simulink model "Intergration"  (R2018b)
settings: Solver=FixedStepDiscrete  StartTime=0.0  StopTime=inf  FixedStep=0.005  RelTol=1e-3
PostLoadFcn:
  | if any(exist('dsrtsu_mdlpostloadfcn', 'file') ~= 0), dsrtsu_mdlpostloadfcn('Execute', bdroot); end
values from neighbouring files (symbols this model uses):
  P_x165_On = 1.0    [CAN_Tx.sldd]
  P_x242_On = 1.0    [CAN_Tx.sldd]
  P_x246_On = 1.0    [CAN_Tx.sldd]
libraries: rtican x112, simulink x59
(part 27 of 31)

== system Intergration/TX/YRS1_0x131 ==
  <VehDynYawRate> : Inport
  In2 : Inport  Port=2
  Cast To Double{1..4} (4 alike) : DataTypeConversion  OutDataTypeStr=double
  Constant : Constant  Value=0  OutDataTypeStr=uint8
  Constant2 : Constant  Value=0  OutDataTypeStr=double
  Constant6 : Constant  Value=7  OutDataTypeStr=uint8
  RollingCounter1 : Subsystem
  S-Function Builder1 : S-Function  InitFcn=try, set_param(gcb,'FunctionName','CheckSum_Tx_Radar410'), end  FunctionName=CheckSum_Tx_Radar410  SFunctionModules=CheckSum_Tx_Radar410_wrapper  SFunctionDeploymentMode=off  EnableBusSupport=off  mask(S-Function Builder){}
      mask help: Simulink:masks:SFunctionBuilder_MD
      mask init: same as Intergration/Tx_410_10ms/S-Function Builder1
      settings: CopyFcn=set_param(gcbh,'LinkStatus','none')  PreSaveFcn=try, set_param(gcb,'FunctionName','CheckSum_Tx_Radar410'), end  OpenFcn=sfunctionwizard(gcbh)
      mask Display: plot(val(:,1),val(:,2)),disp(sys), port_label('input',1,'data'), port_label('input',2,'length'), port_label('output',1,'u8_crc8')
  Subsystem : Subsystem
  Subsystem1 : Subsystem
  Subsystem4 : Subsystem
  Vector Concatenate1 : Concatenate  NumInputs=7
  YRS1 : rtican/RTICAN Transmit (TX)   Reserved1=[]  Reserved2=[]  Reserved3=[]  Reserved4=[]  SfcnMessage=[]  Msg_Struct=[]  BoardTypeNo=[]  BoardNo=[]  ChannelNo=[]  Parameters=[]  DialogFcn=[]  UnitName=[]  Revision=[]  UnitValues=[]  DSProperties=struct('RTI',struct('Version',uint32(5),'BlockType',struct('isSLSource',uint8(1),'isSLSink',uint8(1),'isHWSource',uint8(0),'isHWSink',uint8(0),'isSetup',uint8(0),'isInline',uint8(1),'isNonInline',uint8(0),'isInterrupt',uint8(0),'isChannelwise',uint8(0)),'IOBoardType','RTICAN','UnitType','MESSAGE','Identifier','TX','DialogType','MSVC','BlockSet','RTICAN','SlaveProcessor','CAN'))  RTIBlockInterface=struct('InputPortsWidth',int32([1 1 1 1 1 1]),'InputPortsActive',[1 1 1 1 1 1],'InputPortsName',{{'YRS1_AliveCounter','YRS_YawRate','YRS_LateralAcce','YRS_YawRateSensorState','YRS_LateralSensorState','YRS1_Checksum'}},'InputPortsDataType',{{'SS_DOUBLE','SS_DOUBLE','SS_DOUBLE','SS_DOUBLE','SS_DOUBLE','SS_DOUBLE'}},'OutputPortsWidth',int32([1 1 1 1]),'OutputPortsActive',[1 1 1 1],'OutputPortsName',{{['TX status'],['TX time'],['TX delta time'],['TX delay time']}},'DialogFcn','rtican_message_interface_gui','BlockDisplay',{{'','center'}},'IconTransparency','on','InitLevel',3,'BlockName',struct('Token',{{'YRS1'}}),'SampleTime',{{-1}},'TriggerPort',{{'none'}},'EnablePort',{{'none'}})  RTIBlockParameters=struct('BoardTypeNo',{{1,'OFF',[]}},'BoardNo',{{3,'ON',[1 16]}},'ChannelNo',{{2,'ON',[1 2]}},'Parameters',{{struct('DataFileSupport',struct('DataFileSelectedMaster',1,'DataFileSelectedLocal',1,'DataFileName','c:\users\administrator.zx-201607042142\documents\matlab\zone\dbc\ars410od_privatecan.dbc|c:\users\administrator.zx-201607042142\desktop\zone\2020_demo\410\asr410od_public_can.dbc|','DataFileDate',{{{''},{['30-十一月-2020 09:38:41']}}},'SelectedFile','..\..\..\..\..\desktop\zone\2020_demo\410\asr410od_public_can.dbc','InterfaceFcn','rtican_dbc_file_parser'),'Options',struct('StatusSelected',1,'TimeSelected',1,'DeltaTimeSelected',1,'DelayTimeSelected',1,'DelayTimeTXCommandSelected',0,'EncodeSetUnusedBitsToOne',0,'EnableMsgLoopback',0,'TriggerPort',struct('Selected',0,'TriggerType',0),'EnablePortSelected',0,'SignalOnPortnameSelected',1,'UserCoding',struct('Selected',0,'InterfaceFile','UserEncodingFile','FcnName','UserEncodeFcn','InportSelected',0,'InportWidth',1,'OutportSelected',0,'OutportWidth',1),'TerminationMsg',struct('Selected',0,'Byte0_7','0'),'InitialMsg',struct('Selected',0,'Byte0_7','0')),'Message',struct('MsgOnBlocknameSelected',1,'MsgName','YRS1','MsgIdFormat',0,'MsgId',305,'MsgLength',8,'NumSignals',6,'SampleTime',-1,'StartTime',struct('Selected',0,'Value',3),'AutoRepeatTime',struct('Selected',0,'Value',0.1),'Timeout',struct('Selected',0,'Value',0.1),'DelayTime',struct('Selected',0,'Value',0.1),'Signal',struct('SgnName',{'YRS1_AliveCounter','YRS_YawRate','YRS_LateralAcce','YRS_YawRateSensorState','YRS_LateralSensorState','YRS1_Checksum'},'SgnStartBit',{0,16,32,49,51,56},'SgnLength',{4,16,16,2,2,8},'SgnType',{0,0,0,0,0,0},'ModeValue',{-1,-1,-1,-1,-1,-1},'DataType',{0,0,0,0,0,0},'ByteLayout',{2,2,2,2,2,2},'Factor',{1,0.01,0.001,1,1,1},'Offset',{0,-180,-2,0,0,0},'SgnComment',{{'YRS1_AliveCounter'},{'YRS_YawRate'},{'YRS_LateralAcce'},{'YRS_YawRateSensorState'},{'YRS_LateralSensorState'},{'YRS1_Checksum'}},'SgnUnit',{'','','','','',''},'Min',{0,-180,-2,0,0,0},'Max',{15,180,2,3,3,255},'SLDataType',{'SS_DOUBLE','SS_DOUBLE','SS_DOUBLE','SS_DOUBLE','SS_DOUBLE','SS_DOUBLE'}),'MsgIdNumFormat',1,'MsgComment',{{''}}),'Version',1.2,'general',struct('isFromLib',0)),'OFF',[]}},'GroupId',{{struct('Group',{{'RTICAN'}},'No',3,'Behavior',{{'NAMECHANGE'}},'BlockType',{{'SINK'}},'NameChangeFlag',0),'OFF',[]}},'SFcnRTICANMessage',{{struct('MsgType','TX','SFcnPortType','Scalar','MsgName','YRS1','MsgIdFormat','STD','MsgId',305,'MsgLength',8,'NumSignals',6,'SampleTime',-1,'StartTime',struct('Selected','no','Value',3),'AutoRepeatTime',struct('Selected','no','Value',0.1),'Timeout',struct('Selected','no','Value',0.1),'Signal',struct('SgnName',{'YRS1_AliveCounter','YRS_YawRate','YRS_LateralAcce','YRS_YawRateSensorState','YRS_LateralSensorState','YRS1_Checksum'},'SgnStartBit',{0,16,32,49,51,56},'SgnLength',{4,16,16,2,2,8},'SgnType',{'standard','standard','standard','standard','standard','standard'},'ModeValue',{-1,-1,-1,-1,-1,-1},'DataType',{['unsigned int'],['unsigned int'],['unsigned int'],['unsigned int'],['unsigned int'],['unsigned int']},'ByteLayout',{['motorola back.'],['motorola back.'],['motorola back.'],['motorola back.'],['motorola back.'],['motorola back.']},'Factor',{1,0.01,0.001,1,1,1},'Offset',{0,-180,-2,0,0,0},'SLDataType',{'SS_DOUBLE','SS_DOUBLE','SS_DOUBLE','SS_DOUBLE','SS_DOUBLE','SS_DOUBLE'}),'StatusSelected','yes','TimeSelected','yes','DeltaTimeSelected','yes','DelayTimeSelected','yes','DelayTimeTXCommandSelected','no','EncodeSetUnusedBitsToOne','no','EnableMsgLoopback','no','TriggerPort',struct('Selected','no','TriggerType',0),'EnablePortSelected','no','UserCoding',struct('Selected','no','InterfaceFile','UserEncodingFile','FcnName','UserEncodeFcn','InportSelected','no','InportWidth',1,'OutportSelected','no','OutportWidth',1),'TerminationMsg',struct('Selected','no','Byte0','0x00','Byte1','0x00','Byte2','0x00','Byte3','0x00','Byte4','0x00','Byte5','0x00','Byte6','0x00','Byte7','0x00'),'InitialMsg',struct('Selected','no','Byte0','0x00','Byte1','0x00','Byte2','0x00','Byte3','0x00','Byte4','0x00','Byte5','0x00','Byte6','0x00','Byte7','0x00'),'BoardType','DS1','BoardNo',3,'ControllerNo',2),'OFF',[]}},'TLCFileName',{{'rtican_tx_message','OFF',[]}})  RTISFcnParameters=struct('SFcnRTICANMessage','struct','TLCFileName','char')  RTIBlockParaDefault=struct('BoardTypeNo',4302,'BoardNo',1,'ChannelNo',1,'Parameters',struct('DataFileSupport',struct('DataFileSelectedMaster',0,'DataFileSelectedLocal',0,'DataFileName','','DataFileDate','','SelectedFile',['<no file selected>']),'Options',struct('StatusSelected',1,'TimeSelected',1,'DeltaTimeSelected',1,'DelayTimeSelected',1,'DelayTimeTXCommandSelected',0,'EncodeSetUnusedBitsToOne',0,'EnableMsgLoopback',0,'TriggerPort',struct('Selected',0,'TriggerType','rising'),'EnablePortSelected',0,'SignalOnPortnameSelected',1,'UserCoding',struct('Selected',0,'InterfaceFile','UserEncodingFile','FcnName','UserEncodeFcn','InportSelected',0,'InportWidth',1,'OutportSelected',0,'OutportWidth',1),'TerminationMsg',struct('Selected',0,'Byte0_7','0'),'InitialMsg',struct('Selected',0,'Byte0_7','0')),'Message',struct('MsgOnBlocknameSelected',0,'MsgName',['TX Message'],'MsgIdFormat',0,'MsgId',100,'MsgLength',8,'NumSignals',1,'SampleTime',-1,'StartTime',struct('Selected',0,'Value',0),'AutoRepeatTime',struct('Selected',0,'Value',0.1),'Timeout',struct('Selected',0,'Value',0.1),'DelayTime',struct('Selected',0,'Value',0.1),'Signal',struct('SgnName',['TX signal'],'SgnStartBit',0,'SgnLength',8,'SgnType',0,'ModeValue',-1,'DataType',0,'SLDataType','SS_DOUBLE','ByteLayout',0,'Factor',1,'Offset',0,'Min',0,'Max',255,'SgnComment',{{}},'SgnUnit',''),'MsgIdNumFormat',0,'MsgComment',{{''}}),'Version',1.2,'general',struct('isFromLib',1)),'GroupId',struct('Group',{{'RTICAN'}},'No',1,'Behavior',{{'NAMECHANGE'}},'BlockType',{{'SINK'}},'NameChangeFlag',0),'SFcnRTICANMessage',struct('MsgType','TX','MsgName',['TX Message'],'MsgIdFormat','STD','MsgId',100,'MsgLength',2,'NumSignals',1,'SampleTime',-1,'StartTime',struct('Selected','no','Value',0),'AutoRepeatTime',struct('Selected','no','Value',0.1),'Timeout',struct('Selected','no','Value',0.1),'DelayTime',struct('Selected','no','Value',0.1),'Signal',struct('SgnName',['TX signal'],'SgnStartBit',0,'SgnLength',8,'SgnType','standard','ModeValue',-1,'DataType',['unsigned int'],'ByteLayout',['little endian'],'SLDataType','SS_DOUBLE','Factor',1,'Offset',0),'StatusSelected','yes','TimeSelected','yes','DeltaTimeSelected','yes','DelayTimeSelected','yes','EnablePortSelected','no','EnableMsgLoopback','no','DelayTimeTXCommandSelected','no','EncodeSetUnusedBitsToOne','no','UserCoding',struct('Selected','no','InterfaceFile','UserDecodingFile','FcnName','UserDecodeFcn','InportSelected','no','InportWidth',1,'OutportSelected','no','OutportWidth',1),'TerminationMsg',struct('Selected','no','Byte0','0x00','Byte1','0x00','Byte2','0x00','Byte3','0x00','Byte4','0x00','Byte5','0x00','Byte6','0x00','Byte7','0x00'),'InitialMsg',struct('Selected','no','Byte0','0x00','Byte1','0x00','Byte2','0x00','Byte3','0x00','Byte4','0x00','Byte5','0x00','Byte6','0x00','Byte7','0x00'),'TriggerPort',struct('Selected','no','TriggerType','rising'),'BoardType','DS4302','BoardNo',1,'ControllerNo',1,'SFcnPortType','Scalar'),'TLCFileName','rtican_tx_message')
      settings: AttributesFormatString=Group Id: RTICAN3\n  SourceProductName=dSPACE RTI CAN Blockset
  wires:
  Subsystem1/1(Byte4) -> Vector Concatenate1/3
  Subsystem1/3(Byte5) -> Vector Concatenate1/4
  Subsystem/3(Byte3) -> Vector Concatenate1/2
  Subsystem/1(Byte2) -> Vector Concatenate1/1
  Constant2/1 -> YRS1/5, YRS1/4
  Subsystem1/2(Out2) -> Cast To Double3/1
  Cast To Double2/1 -> YRS1/6
  RollingCounter1/1(RC) -> Cast To Double4/1, Subsystem4/1(In1)
  Cast To Double4/1 -> YRS1/1
  Subsystem4/1(Byte6) -> Vector Concatenate1/5
  Cast To Double1/1 -> YRS1/3
  Constant6/1 -> S-Function Builder1/2
  Cast To Double3/1 -> YRS1/2
  Subsystem/2(Out2) -> Cast To Double1/1
  S-Function Builder1/1 -> Cast To Double2/1
  Vector Concatenate1/1 -> S-Function Builder1/1
  <VehDynYawRate>/1 -> Subsystem1/1(In1)
  In2/1 -> Subsystem/1(In1)
  Constant/1 -> Vector Concatenate1/7, Vector Concatenate1/6

== system Intergration/TX/YRS2_0x132 ==
  In1 : Inport
  Cast To Double1 : DataTypeConversion  OutDataTypeStr=double
  Cast To Double2 : DataTypeConversion  OutDataTypeStr=double
  Cast To Double3 : DataTypeConversion  OutDataTypeStr=double
  Constant : Constant  Value=0  OutDataTypeStr=uint8
  Constant1 : Constant  Value=0  OutDataTypeStr=double
  Constant6 : Constant  Value=7  OutDataTypeStr=uint8
  RollingCounter1 : Subsystem
  S-Function Builder1 : S-Function  InitFcn=try, set_param(gcb,'FunctionName','CheckSum_Tx_Radar410'), end  FunctionName=CheckSum_Tx_Radar410  SFunctionModules=CheckSum_Tx_Radar410_wrapper  SFunctionDeploymentMode=off  EnableBusSupport=off  mask(S-Function Builder){}
      mask help: Simulink:masks:SFunctionBuilder_MD
      mask init: same as Intergration/Tx_410_10ms/S-Function Builder1
      settings: CopyFcn=set_param(gcbh,'LinkStatus','none')  PreSaveFcn=try, set_param(gcb,'FunctionName','CheckSum_Tx_Radar410'), end  OpenFcn=sfunctionwizard(gcbh)
      mask Display: plot(val(:,1),val(:,2)),disp(sys), port_label('input',1,'data'), port_label('input',2,'length'), port_label('output',1,'u8_crc8')
  Subsystem : Subsystem
  Subsystem4 : Subsystem
  Vector Concatenate1 : Concatenate  NumInputs=7
  YRS2 : rtican/RTICAN Transmit (TX)   Reserved1=[]  Reserved2=[]  Reserved3=[]  Reserved4=[]  SfcnMessage=[]  Msg_Struct=[]  BoardTypeNo=[]  BoardNo=[]  ChannelNo=[]  Parameters=[]  DialogFcn=[]  UnitName=[]  Revision=[]  UnitValues=[]  DSProperties=struct('RTI',struct('Version',uint32(5),'BlockType',struct('isSLSource',uint8(1),'isSLSink',uint8(1),'isHWSource',uint8(0),'isHWSink',uint8(0),'isSetup',uint8(0),'isInline',uint8(1),'isNonInline',uint8(0),'isInterrupt',uint8(0),'isChannelwise',uint8(0)),'IOBoardType','RTICAN','UnitType','MESSAGE','Identifier','TX','DialogType','MSVC','BlockSet','RTICAN','SlaveProcessor','CAN'))  RTIBlockInterface=struct('InputPortsWidth',int32([1 1 1 1]),'InputPortsActive',[1 1 1 1],'InputPortsName',{{'YRS_AliveCounter','YRS_LongitAcce','YRS_LongitSensorState','YRS2_Checksum'}},'InputPortsDataType',{{'SS_DOUBLE','SS_DOUBLE','SS_DOUBLE','SS_DOUBLE'}},'OutputPortsWidth',int32([1 1 1 1]),'OutputPortsActive',[1 1 1 1],'OutputPortsName',{{['TX status'],['TX time'],['TX delta time'],['TX delay time']}},'DialogFcn','rtican_message_interface_gui','BlockDisplay',{{'','center'}},'IconTransparency','on','InitLevel',3,'BlockName',struct('Token',{{'YRS2'}}),'SampleTime',{{-1}},'TriggerPort',{{'none'}},'EnablePort',{{'none'}})  RTIBlockParameters=struct('BoardTypeNo',{{1,'OFF',[]}},'BoardNo',{{3,'ON',[1 16]}},'ChannelNo',{{2,'ON',[1 2]}},'Parameters',{{struct('DataFileSupport',struct('DataFileSelectedMaster',1,'DataFileSelectedLocal',1,'DataFileName','c:\users\administrator.zx-201607042142\documents\matlab\zone\dbc\ars410od_privatecan.dbc|c:\users\administrator.zx-201607042142\desktop\zone\2020_demo\410\asr410od_public_can.dbc|','DataFileDate',{{{''},{['30-十一月-2020 09:38:41']}}},'SelectedFile','..\..\..\..\..\desktop\zone\2020_demo\410\asr410od_public_can.dbc','InterfaceFcn','rtican_dbc_file_parser'),'Options',struct('StatusSelected',1,'TimeSelected',1,'DeltaTimeSelected',1,'DelayTimeSelected',1,'DelayTimeTXCommandSelected',0,'EncodeSetUnusedBitsToOne',0,'EnableMsgLoopback',0,'TriggerPort',struct('Selected',0,'TriggerType',0),'EnablePortSelected',0,'SignalOnPortnameSelected',1,'UserCoding',struct('Selected',0,'InterfaceFile','UserEncodingFile','FcnName','UserEncodeFcn','InportSelected',0,'InportWidth',1,'OutportSelected',0,'OutportWidth',1),'TerminationMsg',struct('Selected',0,'Byte0_7','0'),'InitialMsg',struct('Selected',0,'Byte0_7','0')),'Message',struct('MsgOnBlocknameSelected',1,'MsgName','YRS2','MsgIdFormat',0,'MsgId',306,'MsgLength',8,'NumSignals',4,'SampleTime',-1,'StartTime',struct('Selected',0,'Value',3),'AutoRepeatTime',struct('Selected',0,'Value',0.1),'Timeout',struct('Selected',0,'Value',0.1),'DelayTime',struct('Selected',0,'Value',0.1),'Signal',struct('SgnName',{'YRS_AliveCounter','YRS_LongitAcce','YRS_LongitSensorState','YRS2_Checksum'},'SgnStartBit',{0,32,54,56},'SgnLength',{4,16,2,8},'SgnType',{0,0,0,0},'ModeValue',{-1,-1,-1,-1},'DataType',{0,0,0,0},'ByteLayout',{2,2,2,2},'Factor',{1,0.001,1,1},'Offset',{0,-2,0,0},'SgnComment',{{'YRS_AliveCounter'},{'YRS_LongitAcce'},{'YRS_LongitSensorState'},{'YRS2_Checksum'}},'SgnUnit',{'','','',''},'Min',{0,-2,0,0},'Max',{15,2,3,255},'SLDataType',{'SS_DOUBLE','SS_DOUBLE','SS_DOUBLE','SS_DOUBLE'}),'MsgIdNumFormat',1,'MsgComment',{{''}}),'Version',1.2,'general',struct('isFromLib',0)),'OFF',[]}},'GroupId',{{struct('Group',{{'RTICAN'}},'No',3,'Behavior',{{'NAMECHANGE'}},'BlockType',{{'SINK'}},'NameChangeFlag',0),'OFF',[]}},'SFcnRTICANMessage',{{struct('MsgType','TX','SFcnPortType','Scalar','MsgName','YRS2','MsgIdFormat','STD','MsgId',306,'MsgLength',8,'NumSignals',4,'SampleTime',-1,'StartTime',struct('Selected','no','Value',3),'AutoRepeatTime',struct('Selected','no','Value',0.1),'Timeout',struct('Selected','no','Value',0.1),'Signal',struct('SgnName',{'YRS_AliveCounter','YRS_LongitAcce','YRS_LongitSensorState','YRS2_Checksum'},'SgnStartBit',{0,32,54,56},'SgnLength',{4,16,2,8},'SgnType',{'standard','standard','standard','standard'},'ModeValue',{-1,-1,-1,-1},'DataType',{['unsigned int'],['unsigned int'],['unsigned int'],['unsigned int']},'ByteLayout',{['motorola back.'],['motorola back.'],['motorola back.'],['motorola back.']},'Factor',{1,0.001,1,1},'Offset',{0,-2,0,0},'SLDataType',{'SS_DOUBLE','SS_DOUBLE','SS_DOUBLE','SS_DOUBLE'}),'StatusSelected','yes','TimeSelected','yes','DeltaTimeSelected','yes','DelayTimeSelected','yes','DelayTimeTXCommandSelected','no','EncodeSetUnusedBitsToOne','no','EnableMsgLoopback','no','TriggerPort',struct('Selected','no','TriggerType',0),'EnablePortSelected','no','UserCoding',struct('Selected','no','InterfaceFile','UserEncodingFile','FcnName','UserEncodeFcn','InportSelected','no','InportWidth',1,'OutportSelected','no','OutportWidth',1),'TerminationMsg',struct('Selected','no','Byte0','0x00','Byte1','0x00','Byte2','0x00','Byte3','0x00','Byte4','0x00','Byte5','0x00','Byte6','0x00','Byte7','0x00'),'InitialMsg',struct('Selected','no','Byte0','0x00','Byte1','0x00','Byte2','0x00','Byte3','0x00','Byte4','0x00','Byte5','0x00','Byte6','0x00','Byte7','0x00'),'BoardType','DS1','BoardNo',3,'ControllerNo',2),'OFF',[]}},'TLCFileName',{{'rtican_tx_message','OFF',[]}})  RTISFcnParameters=struct('SFcnRTICANMessage','struct','TLCFileName','char')  RTIBlockParaDefault=struct('BoardTypeNo',4302,'BoardNo',1,'ChannelNo',1,'Parameters',struct('DataFileSupport',struct('DataFileSelectedMaster',0,'DataFileSelectedLocal',0,'DataFileName','','DataFileDate','','SelectedFile',['<no file selected>']),'Options',struct('StatusSelected',1,'TimeSelected',1,'DeltaTimeSelected',1,'DelayTimeSelected',1,'DelayTimeTXCommandSelected',0,'EncodeSetUnusedBitsToOne',0,'EnableMsgLoopback',0,'TriggerPort',struct('Selected',0,'TriggerType','rising'),'EnablePortSelected',0,'SignalOnPortnameSelected',1,'UserCoding',struct('Selected',0,'InterfaceFile','UserEncodingFile','FcnName','UserEncodeFcn','InportSelected',0,'InportWidth',1,'OutportSelected',0,'OutportWidth',1),'TerminationMsg',struct('Selected',0,'Byte0_7','0'),'InitialMsg',struct('Selected',0,'Byte0_7','0')),'Message',struct('MsgOnBlocknameSelected',0,'MsgName',['TX Message'],'MsgIdFormat',0,'MsgId',100,'MsgLength',8,'NumSignals',1,'SampleTime',-1,'StartTime',struct('Selected',0,'Value',0),'AutoRepeatTime',struct('Selected',0,'Value',0.1),'Timeout',struct('Selected',0,'Value',0.1),'DelayTime',struct('Selected',0,'Value',0.1),'Signal',struct('SgnName',['TX signal'],'SgnStartBit',0,'SgnLength',8,'SgnType',0,'ModeValue',-1,'DataType',0,'SLDataType','SS_DOUBLE','ByteLayout',0,'Factor',1,'Offset',0,'Min',0,'Max',255,'SgnComment',{{}},'SgnUnit',''),'MsgIdNumFormat',0,'MsgComment',{{''}}),'Version',1.2,'general',struct('isFromLib',1)),'GroupId',struct('Group',{{'RTICAN'}},'No',1,'Behavior',{{'NAMECHANGE'}},'BlockType',{{'SINK'}},'NameChangeFlag',0),'SFcnRTICANMessage',struct('MsgType','TX','MsgName',['TX Message'],'MsgIdFormat','STD','MsgId',100,'MsgLength',2,'NumSignals',1,'SampleTime',-1,'StartTime',struct('Selected','no','Value',0),'AutoRepeatTime',struct('Selected','no','Value',0.1),'Timeout',struct('Selected','no','Value',0.1),'DelayTime',struct('Selected','no','Value',0.1),'Signal',struct('SgnName',['TX signal'],'SgnStartBit',0,'SgnLength',8,'SgnType','standard','ModeValue',-1,'DataType',['unsigned int'],'ByteLayout',['little endian'],'SLDataType','SS_DOUBLE','Factor',1,'Offset',0),'StatusSelected','yes','TimeSelected','yes','DeltaTimeSelected','yes','DelayTimeSelected','yes','EnablePortSelected','no','EnableMsgLoopback','no','DelayTimeTXCommandSelected','no','EncodeSetUnusedBitsToOne','no','UserCoding',struct('Selected','no','InterfaceFile','UserDecodingFile','FcnName','UserDecodeFcn','InportSelected','no','InportWidth',1,'OutportSelected','no','OutportWidth',1),'TerminationMsg',struct('Selected','no','Byte0','0x00','Byte1','0x00','Byte2','0x00','Byte3','0x00','Byte4','0x00','Byte5','0x00','Byte6','0x00','Byte7','0x00'),'InitialMsg',struct('Selected','no','Byte0','0x00','Byte1','0x00','Byte2','0x00','Byte3','0x00','Byte4','0x00','Byte5','0x00','Byte6','0x00','Byte7','0x00'),'TriggerPort',struct('Selected','no','TriggerType','rising'),'BoardType','DS4302','BoardNo',1,'ControllerNo',1,'SFcnPortType','Scalar'),'TLCFileName','rtican_tx_message')
      settings: AttributesFormatString=Group Id: RTICAN3\n  SourceProductName=dSPACE RTI CAN Blockset
  wires:
  In1/1 -> Subsystem/1(In1)
  Constant6/1 -> S-Function Builder1/2
  Subsystem/1(Byte2) -> Vector Concatenate1/1
  Cast To Double2/1 -> YRS2/2
  RollingCounter1/1(RC) -> Subsystem4/1(In1), Cast To Double1/1
  Subsystem/3(Byte3) -> Vector Concatenate1/2
  Vector Concatenate1/1 -> S-Function Builder1/1
  Cast To Double1/1 -> YRS2/1
  Cast To Double3/1 -> YRS2/4
  Subsystem/2(Out2) -> Cast To Double2/1
  Constant1/1 -> YRS2/3
  Subsystem4/1(Byte6) -> Vector Concatenate1/3
  S-Function Builder1/1 -> Cast To Double3/1
  Constant/1 -> Vector Concatenate1/7, Vector Concatenate1/6, Vector Concatenate1/5, Vector Concatenate1/4

== system Intergration/Tx_410_10ms/RollingCounter1 ==
  Add2 : Sum
  Constant5 : Constant
  Constant6 : Constant  Value=-1
  Delay : Delay  DelayLength=1
  Switch : Switch  Criteria=u2 > Threshold  Threshold=14
  RC : Outport
  wires:
  Constant6/1 -> Switch/1
  Switch/1 -> Add2/2
  Delay/1 -> RC/1, Switch/3, Switch/2
  Add2/1 -> Delay/1
  Constant5/1 -> Add2/1

== system Intergration/Tx_410_10ms/Subsystem ==
  In1 : Inport
  Bitwise Operator1 : simulink/Logic and Bit Operations/Bitwise Operator  logicop=AND  UseBitMask=on  BitMask=bin2dec('11111111')  BitMaskRealWorld=Stored Integer
  Data Type Conversion1 : DataTypeConversion  OutDataTypeStr=uint8
  Byte2 : Outport
  wires:
  Data Type Conversion1/1 -> Bitwise Operator1/1
  Bitwise Operator1/1 -> Byte2/1
  In1/1 -> Data Type Conversion1/1

== system Intergration/Tx_410_10ms/Subsystem1 ==
  In1 : Inport
  Add : Sum
  Add1 : Sum  Inputs=+-
  Bitwise Operator1 : simulink/Logic and Bit Operations/Bitwise Operator  logicop=AND  UseBitMask=on  BitMask=bin2dec('11111111')  BitMaskRealWorld=Stored Integer
  Bitwise Operator2 : simulink/Logic and Bit Operations/Bitwise Operator  logicop=AND  UseBitMask=on  BitMask=bin2dec('11111111')  BitMaskRealWorld=Stored Integer
  Constant1 : Constant  Value=780
  Constant2 : Constant  Value=0.1
  Constant3 : Constant  Value=0.1
  Constant4 : Constant  Value=780
  Data Type Conversion1 : DataTypeConversion  OutDataTypeStr=uint16
  Data Type Conversion2 : DataTypeConversion  OutDataTypeStr=uint8
  Data Type Conversion3 : DataTypeConversion  OutDataTypeStr=uint8
  Divide1 : Product  Inputs=*/
  Multiply : Product
  Shift Arithmetic1 : ArithShift  BitShiftNumber=8  BitShiftDirection=Right
  Byte0 : Outport
  Out2 : Outport  Port=2
  Byte1 : Outport  Port=3
  wires:
  Constant2/1 -> Divide1/2
  Constant1/1 -> Add/2
  Data Type Conversion1/1 -> Bitwise Operator2/1, Multiply/1, Shift Arithmetic1/1
  Shift Arithmetic1/1 -> Bitwise Operator1/1
  Constant4/1 -> Add1/2
  Constant3/1 -> Multiply/2
  Multiply/1 -> Add1/1
  Bitwise Operator1/1 -> Data Type Conversion2/1
  Divide1/1 -> Data Type Conversion1/1
  Add/1 -> Divide1/1
  Add1/1 -> Out2/1
  Bitwise Operator2/1 -> Data Type Conversion3/1
  In1/1 -> Add/1
  Data Type Conversion2/1 -> Byte0/1
  Data Type Conversion3/1 -> Byte1/1

== system Intergration/Tx_410_10ms/Subsystem4 ==
  In1 : Inport
  Bitwise Operator2 : simulink/Logic and Bit Operations/Bitwise Operator  logicop=AND  UseBitMask=on  BitMask=bin2dec('11110000')  BitMaskRealWorld=Stored Integer
  Data Type Conversion1 : DataTypeConversion  OutDataTypeStr=uint8
  Shift Arithmetic1 : ArithShift  BitShiftNumber=4  BitShiftDirection=Left
  Byte4 : Outport
  wires:
  In1/1 -> Data Type Conversion1/1
  Bitwise Operator2/1 -> Byte4/1
  Data Type Conversion1/1 -> Shift Arithmetic1/1
  Shift Arithmetic1/1 -> Bitwise Operator2/1

== system Intergration/RTI Data/RTI Data Store/RTI Data Store ==
  RTI Data Store : Subsystem  mask(RTI_DATA_STORE){}
      mask help:
      | RTI Data Store Block. This block is used by RTI to store internal model dependent data. Deleting this block will result in data loss.
      |
      | NEVER DELETE, COPY, OR MODIFY THIS BLOCK!
      mask Help:
      | RTI Data Store Block. This block is used by RTI to store internal model dependent data. Deleting this block will result in data loss.
      | 
      | NEVER DELETE, COPY, OR MODIFY THIS BLOCK!
      mask Display: text(0.5, 0.5, ' ', 'HorizontalAlignment', 'center');

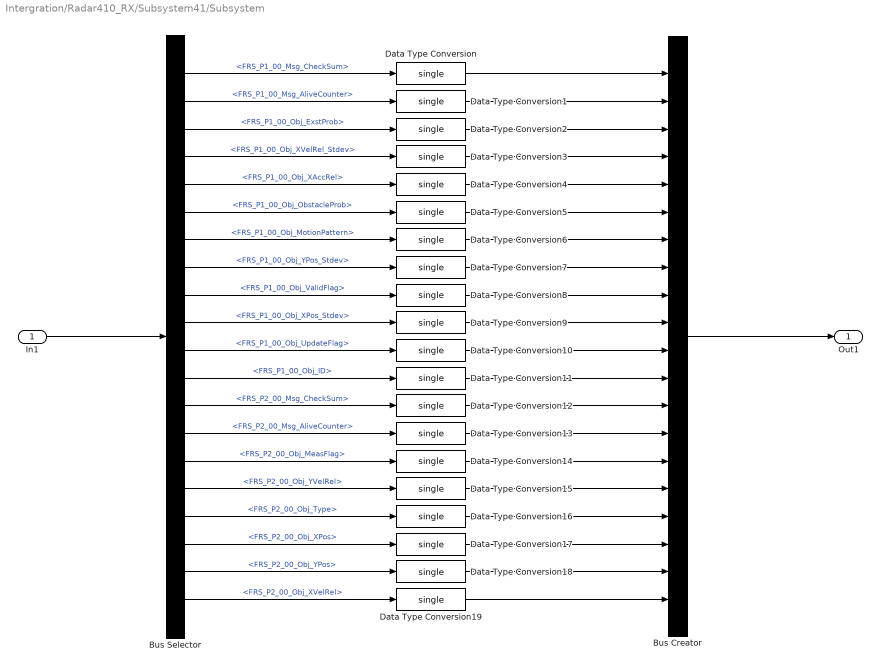
== system Intergration/Radar410_RX/Subsystem41/Subsystem ==
  In1 : Inport
  Bus Creator : BusCreator  Inputs=20  OutDataTypeStr=Bus: Obj_Data  NonVirtualBus=on
      settings: InheritFromInputs=off
  Bus Selector : BusSelector  OutputSignals=FRS_P1_00_Msg_CheckSum,FRS_P1_00_Msg_AliveCounter,FRS_P1_00_Obj_ExstProb,FRS_P1_00_Obj_XVelRel_Stdev,FRS_P1_00_Obj_XAccRel,FRS_P1_00_Obj_ObstacleProb,FRS_P1_00_Obj_MotionPattern,FRS_P1_00_Obj_YPos_Stdev,FRS_P1_00_Obj_ValidFlag,FRS_P1_00_Obj_XPos_Stdev,FRS_P1_00_Obj_UpdateFlag,FRS_P1_00_Obj_ID,FRS_P2_00_Msg_CheckSum,FRS_P2_00_Msg_AliveCounter,FRS_P2_00_Obj_MeasFlag,FRS_P2_00_Obj_YVelRel,FRS_P2_00_Obj_Type,FRS_P2_00_Obj_XPos,FRS_P2_00_Obj_YPos,FRS_P2_00_Obj_XVelRel
  Data Type Conversion{,1..19} (20 alike) : DataTypeConversion  OutDataTypeStr=single
  Out1 : Outport  OutDataTypeStr=Bus: Obj_Data
  wires:
  Data Type Conversion12/1 -> Bus Creator/13
  Bus Selector/5 -> Data Type Conversion4/1  "<FRS_P1_00_Obj_XAccRel>"
  Bus Selector/8 -> Data Type Conversion7/1  "<FRS_P1_00_Obj_YPos_Stdev>"
  Data Type Conversion15/1 -> Bus Creator/16
  Bus Selector/1 -> Data Type Conversion/1  "<FRS_P1_00_Msg_CheckSum>"
  Bus Selector/15 -> Data Type Conversion14/1  "<FRS_P2_00_Obj_MeasFlag>"
  Bus Selector/3 -> Data Type Conversion2/1  "<FRS_P1_00_Obj_ExstProb>"
  Bus Selector/13 -> Data Type Conversion12/1  "<FRS_P2_00_Msg_CheckSum>"
  Bus Selector/2 -> Data Type Conversion1/1  "<FRS_P1_00_Msg_AliveCounter>"
  Data Type Conversion11/1 -> Bus Creator/12
  Data Type Conversion5/1 -> Bus Creator/6
  Bus Selector/4 -> Data Type Conversion3/1  "<FRS_P1_00_Obj_XVelRel_Stdev>"
  Bus Selector/7 -> Data Type Conversion6/1  "<FRS_P1_00_Obj_MotionPattern>"
  Data Type Conversion9/1 -> Bus Creator/10
  Bus Selector/6 -> Data Type Conversion5/1  "<FRS_P1_00_Obj_ObstacleProb>"
  Data Type Conversion18/1 -> Bus Creator/19
  Bus Selector/11 -> Data Type Conversion10/1  "<FRS_P1_00_Obj_UpdateFlag>"
  Data Type Conversion17/1 -> Bus Creator/18
  Bus Selector/16 -> Data Type Conversion15/1  "<FRS_P2_00_Obj_YVelRel>"
  Data Type Conversion6/1 -> Bus Creator/7
  Bus Selector/12 -> Data Type Conversion11/1  "<FRS_P1_00_Obj_ID>"
  Data Type Conversion16/1 -> Bus Creator/17
  Bus Selector/9 -> Data Type Conversion8/1  "<FRS_P1_00_Obj_ValidFlag>"
  Bus Selector/17 -> Data Type Conversion16/1  "<FRS_P2_00_Obj_Type>"
  Bus Selector/10 -> Data Type Conversion9/1  "<FRS_P1_00_Obj_XPos_Stdev>"
  Data Type Conversion10/1 -> Bus Creator/11
  Bus Selector/14 -> Data Type Conversion13/1  "<FRS_P2_00_Msg_AliveCounter>"
  Bus Selector/19 -> Data Type Conversion18/1  "<FRS_P2_00_Obj_YPos>"
  Bus Selector/18 -> Data Type Conversion17/1  "<FRS_P2_00_Obj_XPos>"
  Bus Selector/20 -> Data Type Conversion19/1  "<FRS_P2_00_Obj_XVelRel>"
  In1/1 -> Bus Selector/1
  Bus Creator/1 -> Out1/1
  Data Type Conversion/1 -> Bus Creator/1
  Data Type Conversion2/1 -> Bus Creator/3
  Data Type Conversion13/1 -> Bus Creator/14
  Data Type Conversion1/1 -> Bus Creator/2
  Data Type Conversion4/1 -> Bus Creator/5
  Data Type Conversion3/1 -> Bus Creator/4
  Data Type Conversion7/1 -> Bus Creator/8
  Data Type Conversion8/1 -> Bus Creator/9
  Data Type Conversion14/1 -> Bus Creator/15
  Data Type Conversion19/1 -> Bus Creator/20

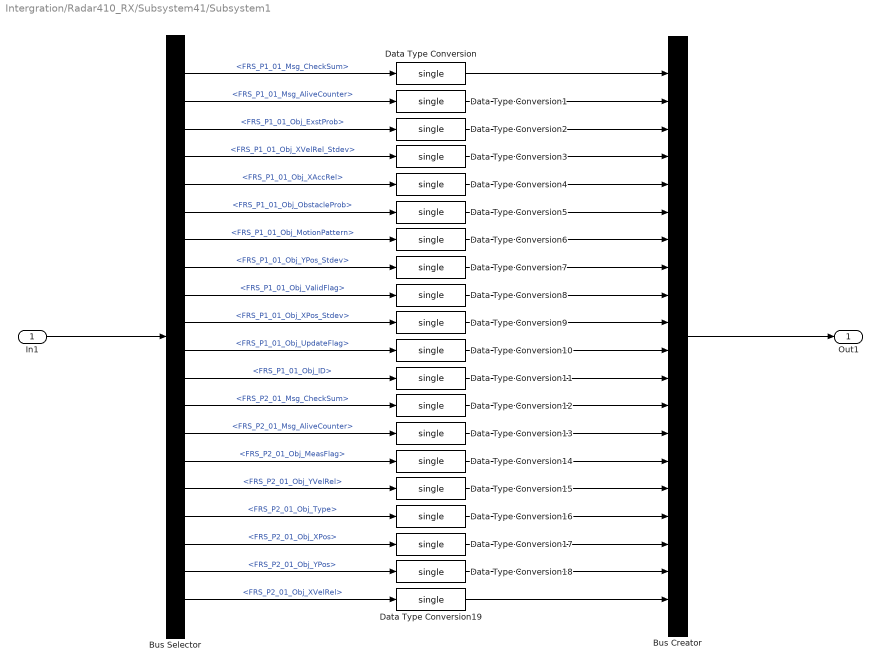
== system Intergration/Radar410_RX/Subsystem41/Subsystem1 ==
  In1 : Inport
  Bus Creator : BusCreator  Inputs=20  OutDataTypeStr=Bus: Obj_Data  NonVirtualBus=on
      settings: InheritFromInputs=off
  Bus Selector : BusSelector  OutputSignals=FRS_P1_01_Msg_CheckSum,FRS_P1_01_Msg_AliveCounter,FRS_P1_01_Obj_ExstProb,FRS_P1_01_Obj_XVelRel_Stdev,FRS_P1_01_Obj_XAccRel,FRS_P1_01_Obj_ObstacleProb,FRS_P1_01_Obj_MotionPattern,FRS_P1_01_Obj_YPos_Stdev,FRS_P1_01_Obj_ValidFlag,FRS_P1_01_Obj_XPos_Stdev,FRS_P1_01_Obj_UpdateFlag,FRS_P1_01_Obj_ID,FRS_P2_01_Msg_CheckSum,FRS_P2_01_Msg_AliveCounter,FRS_P2_01_Obj_MeasFlag,FRS_P2_01_Obj_YVelRel,FRS_P2_01_Obj_Type,FRS_P2_01_Obj_XPos,FRS_P2_01_Obj_YPos,FRS_P2_01_Obj_XVelRel
  Data Type Conversion{,1..19} (20 alike) : DataTypeConversion  OutDataTypeStr=single
  Out1 : Outport  OutDataTypeStr=Bus: Obj_Data
  wires:
  Data Type Conversion19/1 -> Bus Creator/20
  Data Type Conversion14/1 -> Bus Creator/15
  Data Type Conversion8/1 -> Bus Creator/9
  Data Type Conversion7/1 -> Bus Creator/8
  Data Type Conversion3/1 -> Bus Creator/4
  Data Type Conversion4/1 -> Bus Creator/5
  Data Type Conversion1/1 -> Bus Creator/2
  Data Type Conversion13/1 -> Bus Creator/14
  Data Type Conversion2/1 -> Bus Creator/3
  Data Type Conversion/1 -> Bus Creator/1
  Bus Creator/1 -> Out1/1
  In1/1 -> Bus Selector/1
  Bus Selector/20 -> Data Type Conversion19/1  "<FRS_P2_01_Obj_XVelRel>"
  Bus Selector/18 -> Data Type Conversion17/1  "<FRS_P2_01_Obj_XPos>"
  Bus Selector/19 -> Data Type Conversion18/1  "<FRS_P2_01_Obj_YPos>"
  Bus Selector/14 -> Data Type Conversion13/1  "<FRS_P2_01_Msg_AliveCounter>"
  Data Type Conversion10/1 -> Bus Creator/11
  Bus Selector/10 -> Data Type Conversion9/1  "<FRS_P1_01_Obj_XPos_Stdev>"
  Bus Selector/17 -> Data Type Conversion16/1  "<FRS_P2_01_Obj_Type>"
  Bus Selector/9 -> Data Type Conversion8/1  "<FRS_P1_01_Obj_ValidFlag>"
  Data Type Conversion16/1 -> Bus Creator/17
  Bus Selector/12 -> Data Type Conversion11/1  "<FRS_P1_01_Obj_ID>"
  Data Type Conversion6/1 -> Bus Creator/7
  Bus Selector/16 -> Data Type Conversion15/1  "<FRS_P2_01_Obj_YVelRel>"
  Data Type Conversion17/1 -> Bus Creator/18
  Bus Selector/11 -> Data Type Conversion10/1  "<FRS_P1_01_Obj_UpdateFlag>"
  Data Type Conversion18/1 -> Bus Creator/19
  Bus Selector/6 -> Data Type Conversion5/1  "<FRS_P1_01_Obj_ObstacleProb>"
  Data Type Conversion9/1 -> Bus Creator/10
  Bus Selector/7 -> Data Type Conversion6/1  "<FRS_P1_01_Obj_MotionPattern>"
  Bus Selector/4 -> Data Type Conversion3/1  "<FRS_P1_01_Obj_XVelRel_Stdev>"
  Data Type Conversion5/1 -> Bus Creator/6
  Data Type Conversion11/1 -> Bus Creator/12
  Bus Selector/2 -> Data Type Conversion1/1  "<FRS_P1_01_Msg_AliveCounter>"
  Bus Selector/13 -> Data Type Conversion12/1  "<FRS_P2_01_Msg_CheckSum>"
  Bus Selector/3 -> Data Type Conversion2/1  "<FRS_P1_01_Obj_ExstProb>"
  Bus Selector/15 -> Data Type Conversion14/1  "<FRS_P2_01_Obj_MeasFlag>"
  Bus Selector/1 -> Data Type Conversion/1  "<FRS_P1_01_Msg_CheckSum>"
  Data Type Conversion15/1 -> Bus Creator/16
  Bus Selector/8 -> Data Type Conversion7/1  "<FRS_P1_01_Obj_YPos_Stdev>"
  Bus Selector/5 -> Data Type Conversion4/1  "<FRS_P1_01_Obj_XAccRel>"
  Data Type Conversion12/1 -> Bus Creator/13

== system Intergration/Radar410_RX/Subsystem41/Subsystem10 ==
  In1 : Inport
  Bus Creator : BusCreator  Inputs=20  OutDataTypeStr=Bus: Obj_Data  NonVirtualBus=on
      settings: InheritFromInputs=off
  Bus Selector : BusSelector  OutputSignals=FRS_P1_10_Msg_CheckSum,FRS_P1_10_Msg_AliveCounter,FRS_P1_10_Obj_ExstProb,FRS_P1_10_Obj_XVelRel_Stdev,FRS_P1_10_Obj_XAccRel,FRS_P1_10_Obj_ObstacleProb,FRS_P1_10_Obj_MotionPattern,FRS_P1_10_Obj_YPos_Stdev,FRS_P1_10_Obj_ValidFlag,FRS_P1_10_Obj_XPos_Stdev,FRS_P1_10_Obj_UpdateFlag,FRS_P1_10_Obj_ID,FRS_P2_10_Msg_CheckSum,FRS_P2_10_Msg_AliveCounter,FRS_P2_10_Obj_MeasFlag,FRS_P2_10_Obj_YVelRel,FRS_P2_10_Obj_Type,FRS_P2_10_Obj_XPos,FRS_P2_10_Obj_YPos,FRS_P2_10_Obj_XVelRel
  Data Type Conversion{,1..19} (20 alike) : DataTypeConversion  OutDataTypeStr=single
  Out1 : Outport  OutDataTypeStr=Bus: Obj_Data
  wires:
  Data Type Conversion19/1 -> Bus Creator/20
  Data Type Conversion14/1 -> Bus Creator/15
  Data Type Conversion8/1 -> Bus Creator/9
  Data Type Conversion7/1 -> Bus Creator/8
  Data Type Conversion3/1 -> Bus Creator/4
  Data Type Conversion4/1 -> Bus Creator/5
  Data Type Conversion1/1 -> Bus Creator/2
  Data Type Conversion13/1 -> Bus Creator/14
  Data Type Conversion2/1 -> Bus Creator/3
  Data Type Conversion/1 -> Bus Creator/1
  Bus Creator/1 -> Out1/1
  In1/1 -> Bus Selector/1
  Bus Selector/20 -> Data Type Conversion19/1  "<FRS_P2_10_Obj_XVelRel>"
  Bus Selector/18 -> Data Type Conversion17/1  "<FRS_P2_10_Obj_XPos>"
  Bus Selector/19 -> Data Type Conversion18/1  "<FRS_P2_10_Obj_YPos>"
  Bus Selector/14 -> Data Type Conversion13/1  "<FRS_P2_10_Msg_AliveCounter>"
  Data Type Conversion10/1 -> Bus Creator/11
  Bus Selector/10 -> Data Type Conversion9/1  "<FRS_P1_10_Obj_XPos_Stdev>"
  Bus Selector/17 -> Data Type Conversion16/1  "<FRS_P2_10_Obj_Type>"
  Bus Selector/9 -> Data Type Conversion8/1  "<FRS_P1_10_Obj_ValidFlag>"
  Data Type Conversion16/1 -> Bus Creator/17
  Bus Selector/12 -> Data Type Conversion11/1  "<FRS_P1_10_Obj_ID>"
  Data Type Conversion6/1 -> Bus Creator/7
  Bus Selector/16 -> Data Type Conversion15/1  "<FRS_P2_10_Obj_YVelRel>"
  Data Type Conversion17/1 -> Bus Creator/18
  Bus Selector/11 -> Data Type Conversion10/1  "<FRS_P1_10_Obj_UpdateFlag>"
  Data Type Conversion18/1 -> Bus Creator/19
  Bus Selector/6 -> Data Type Conversion5/1  "<FRS_P1_10_Obj_ObstacleProb>"
  Data Type Conversion9/1 -> Bus Creator/10
  Bus Selector/7 -> Data Type Conversion6/1  "<FRS_P1_10_Obj_MotionPattern>"
  Bus Selector/4 -> Data Type Conversion3/1  "<FRS_P1_10_Obj_XVelRel_Stdev>"
  Data Type Conversion5/1 -> Bus Creator/6
  Data Type Conversion11/1 -> Bus Creator/12
  Bus Selector/2 -> Data Type Conversion1/1  "<FRS_P1_10_Msg_AliveCounter>"
  Bus Selector/13 -> Data Type Conversion12/1  "<FRS_P2_10_Msg_CheckSum>"
  Bus Selector/3 -> Data Type Conversion2/1  "<FRS_P1_10_Obj_ExstProb>"
  Bus Selector/15 -> Data Type Conversion14/1  "<FRS_P2_10_Obj_MeasFlag>"
  Bus Selector/1 -> Data Type Conversion/1  "<FRS_P1_10_Msg_CheckSum>"
  Data Type Conversion15/1 -> Bus Creator/16
  Bus Selector/8 -> Data Type Conversion7/1  "<FRS_P1_10_Obj_YPos_Stdev>"
  Bus Selector/5 -> Data Type Conversion4/1  "<FRS_P1_10_Obj_XAccRel>"
  Data Type Conversion12/1 -> Bus Creator/13

== system Intergration/Radar410_RX/Subsystem41/Subsystem11 ==
  In1 : Inport
  Bus Creator : BusCreator  Inputs=20  OutDataTypeStr=Bus: Obj_Data  NonVirtualBus=on
      settings: InheritFromInputs=off
  Bus Selector : BusSelector  OutputSignals=FRS_P1_11_Msg_CheckSum,FRS_P1_11_Msg_AliveCounter,FRS_P1_11_Obj_ExstProb,FRS_P1_11_Obj_XVelRel_Stdev,FRS_P1_11_Obj_XAccRel,FRS_P1_11_Obj_ObstacleProb,FRS_P1_11_Obj_MotionPattern,FRS_P1_11_Obj_YPos_Stdev,FRS_P1_11_Obj_ValidFlag,FRS_P1_11_Obj_XPos_Stdev,FRS_P1_11_Obj_UpdateFlag,FRS_P1_11_Obj_ID,FRS_P2_11_Msg_CheckSum,FRS_P2_11_Msg_AliveCounter,FRS_P2_11_Obj_MeasFlag,FRS_P2_11_Obj_YVelRel,FRS_P2_11_Obj_Type,FRS_P2_11_Obj_XPos,FRS_P2_11_Obj_YPos,FRS_P2_11_Obj_XVelRel
  Data Type Conversion{,1..19} (20 alike) : DataTypeConversion  OutDataTypeStr=single
  Out1 : Outport  OutDataTypeStr=Bus: Obj_Data
  wires:
  Data Type Conversion12/1 -> Bus Creator/13
  Bus Selector/5 -> Data Type Conversion4/1  "<FRS_P1_11_Obj_XAccRel>"
  Bus Selector/8 -> Data Type Conversion7/1  "<FRS_P1_11_Obj_YPos_Stdev>"
  Data Type Conversion15/1 -> Bus Creator/16
  Bus Selector/1 -> Data Type Conversion/1  "<FRS_P1_11_Msg_CheckSum>"
  Bus Selector/15 -> Data Type Conversion14/1  "<FRS_P2_11_Obj_MeasFlag>"
  Bus Selector/3 -> Data Type Conversion2/1  "<FRS_P1_11_Obj_ExstProb>"
  Bus Selector/13 -> Data Type Conversion12/1  "<FRS_P2_11_Msg_CheckSum>"
  Bus Selector/2 -> Data Type Conversion1/1  "<FRS_P1_11_Msg_AliveCounter>"
  Data Type Conversion11/1 -> Bus Creator/12
  Data Type Conversion5/1 -> Bus Creator/6
  Bus Selector/4 -> Data Type Conversion3/1  "<FRS_P1_11_Obj_XVelRel_Stdev>"
  Bus Selector/7 -> Data Type Conversion6/1  "<FRS_P1_11_Obj_MotionPattern>"
  Data Type Conversion9/1 -> Bus Creator/10
  Bus Selector/6 -> Data Type Conversion5/1  "<FRS_P1_11_Obj_ObstacleProb>"
  Data Type Conversion18/1 -> Bus Creator/19
  Bus Selector/11 -> Data Type Conversion10/1  "<FRS_P1_11_Obj_UpdateFlag>"
  Data Type Conversion17/1 -> Bus Creator/18
  Bus Selector/16 -> Data Type Conversion15/1  "<FRS_P2_11_Obj_YVelRel>"
  Data Type Conversion6/1 -> Bus Creator/7
  Bus Selector/12 -> Data Type Conversion11/1  "<FRS_P1_11_Obj_ID>"
  Data Type Conversion16/1 -> Bus Creator/17
  Bus Selector/9 -> Data Type Conversion8/1  "<FRS_P1_11_Obj_ValidFlag>"
  Bus Selector/17 -> Data Type Conversion16/1  "<FRS_P2_11_Obj_Type>"
  Bus Selector/10 -> Data Type Conversion9/1  "<FRS_P1_11_Obj_XPos_Stdev>"
  Data Type Conversion10/1 -> Bus Creator/11
  Bus Selector/14 -> Data Type Conversion13/1  "<FRS_P2_11_Msg_AliveCounter>"
  Bus Selector/19 -> Data Type Conversion18/1  "<FRS_P2_11_Obj_YPos>"
  Bus Selector/18 -> Data Type Conversion17/1  "<FRS_P2_11_Obj_XPos>"
  Bus Selector/20 -> Data Type Conversion19/1  "<FRS_P2_11_Obj_XVelRel>"
  In1/1 -> Bus Selector/1
  Bus Creator/1 -> Out1/1
  Data Type Conversion/1 -> Bus Creator/1
  Data Type Conversion2/1 -> Bus Creator/3
  Data Type Conversion13/1 -> Bus Creator/14
  Data Type Conversion1/1 -> Bus Creator/2
  Data Type Conversion4/1 -> Bus Creator/5
  Data Type Conversion3/1 -> Bus Creator/4
  Data Type Conversion7/1 -> Bus Creator/8
  Data Type Conversion8/1 -> Bus Creator/9
  Data Type Conversion14/1 -> Bus Creator/15
  Data Type Conversion19/1 -> Bus Creator/20

== system Intergration/Radar410_RX/Subsystem41/Subsystem12 ==
  In1 : Inport
  Bus Creator : BusCreator  Inputs=20  OutDataTypeStr=Bus: Obj_Data  NonVirtualBus=on
      settings: InheritFromInputs=off
  Bus Selector : BusSelector  OutputSignals=FRS_P1_12_Msg_CheckSum,FRS_P1_12_Msg_AliveCounter,FRS_P1_12_Obj_ExstProb,FRS_P1_12_Obj_XVelRel_Stdev,FRS_P1_12_Obj_XAccRel,FRS_P1_12_Obj_ObstacleProb,FRS_P1_12_Obj_MotionPattern,FRS_P1_12_Obj_YPos_Stdev,FRS_P1_12_Obj_ValidFlag,FRS_P1_12_Obj_XPos_Stdev,FRS_P1_12_Obj_UpdateFlag,FRS_P1_12_Obj_ID,FRS_P2_12_Msg_CheckSum,FRS_P2_12_Msg_AliveCounter,FRS_P2_12_Obj_MeasFlag,FRS_P2_12_Obj_YVelRel,FRS_P2_12_Obj_Type,FRS_P2_12_Obj_XPos,FRS_P2_12_Obj_YPos,FRS_P2_12_Obj_XVelRel
  Data Type Conversion{,1..19} (20 alike) : DataTypeConversion  OutDataTypeStr=single
  Out1 : Outport  OutDataTypeStr=Bus: Obj_Data
  wires:
  Data Type Conversion19/1 -> Bus Creator/20
  Data Type Conversion14/1 -> Bus Creator/15
  Data Type Conversion8/1 -> Bus Creator/9
  Data Type Conversion7/1 -> Bus Creator/8
  Data Type Conversion3/1 -> Bus Creator/4
  Data Type Conversion4/1 -> Bus Creator/5
  Data Type Conversion1/1 -> Bus Creator/2
  Data Type Conversion13/1 -> Bus Creator/14
  Data Type Conversion2/1 -> Bus Creator/3
  Data Type Conversion/1 -> Bus Creator/1
  Bus Creator/1 -> Out1/1
  In1/1 -> Bus Selector/1
  Bus Selector/20 -> Data Type Conversion19/1  "<FRS_P2_12_Obj_XVelRel>"
  Bus Selector/18 -> Data Type Conversion17/1  "<FRS_P2_12_Obj_XPos>"
  Bus Selector/19 -> Data Type Conversion18/1  "<FRS_P2_12_Obj_YPos>"
  Bus Selector/14 -> Data Type Conversion13/1  "<FRS_P2_12_Msg_AliveCounter>"
  Data Type Conversion10/1 -> Bus Creator/11
  Bus Selector/10 -> Data Type Conversion9/1  "<FRS_P1_12_Obj_XPos_Stdev>"
  Bus Selector/17 -> Data Type Conversion16/1  "<FRS_P2_12_Obj_Type>"
  Bus Selector/9 -> Data Type Conversion8/1  "<FRS_P1_12_Obj_ValidFlag>"
  Data Type Conversion16/1 -> Bus Creator/17
  Bus Selector/12 -> Data Type Conversion11/1  "<FRS_P1_12_Obj_ID>"
  Data Type Conversion6/1 -> Bus Creator/7
  Bus Selector/16 -> Data Type Conversion15/1  "<FRS_P2_12_Obj_YVelRel>"
  Data Type Conversion17/1 -> Bus Creator/18
  Bus Selector/11 -> Data Type Conversion10/1  "<FRS_P1_12_Obj_UpdateFlag>"
  Data Type Conversion18/1 -> Bus Creator/19
  Bus Selector/6 -> Data Type Conversion5/1  "<FRS_P1_12_Obj_ObstacleProb>"
  Data Type Conversion9/1 -> Bus Creator/10
  Bus Selector/7 -> Data Type Conversion6/1  "<FRS_P1_12_Obj_MotionPattern>"
  Bus Selector/4 -> Data Type Conversion3/1  "<FRS_P1_12_Obj_XVelRel_Stdev>"
  Data Type Conversion5/1 -> Bus Creator/6
  Data Type Conversion11/1 -> Bus Creator/12
  Bus Selector/2 -> Data Type Conversion1/1  "<FRS_P1_12_Msg_AliveCounter>"
  Bus Selector/13 -> Data Type Conversion12/1  "<FRS_P2_12_Msg_CheckSum>"
  Bus Selector/3 -> Data Type Conversion2/1  "<FRS_P1_12_Obj_ExstProb>"
  Bus Selector/15 -> Data Type Conversion14/1  "<FRS_P2_12_Obj_MeasFlag>"
  Bus Selector/1 -> Data Type Conversion/1  "<FRS_P1_12_Msg_CheckSum>"
  Data Type Conversion15/1 -> Bus Creator/16
  Bus Selector/8 -> Data Type Conversion7/1  "<FRS_P1_12_Obj_YPos_Stdev>"
  Bus Selector/5 -> Data Type Conversion4/1  "<FRS_P1_12_Obj_XAccRel>"
  Data Type Conversion12/1 -> Bus Creator/13

== system Intergration/Radar410_RX/Subsystem41/Subsystem13 ==
  In1 : Inport
  Bus Creator : BusCreator  Inputs=20  OutDataTypeStr=Bus: Obj_Data  NonVirtualBus=on
      settings: InheritFromInputs=off
  Bus Selector : BusSelector  OutputSignals=FRS_P1_13_Msg_CheckSum,FRS_P1_13_Msg_AliveCounter,FRS_P1_13_Obj_ExstProb,FRS_P1_13_Obj_XVelRel_Stdev,FRS_P1_13_Obj_XAccRel,FRS_P1_13_Obj_ObstacleProb,FRS_P1_13_Obj_MotionPattern,FRS_P1_13_Obj_YPos_Stdev,FRS_P1_13_Obj_ValidFlag,FRS_P1_13_Obj_XPos_Stdev,FRS_P1_13_Obj_UpdateFlag,FRS_P1_13_Obj_ID,FRS_P2_13_Msg_CheckSum,FRS_P2_13_Msg_AliveCounter,FRS_P2_13_Obj_MeasFlag,FRS_P2_13_Obj_YVelRel,FRS_P2_13_Obj_Type,FRS_P2_13_Obj_XPos,FRS_P2_13_Obj_YPos,FRS_P2_13_Obj_XVelRel
  Data Type Conversion{,1..19} (20 alike) : DataTypeConversion  OutDataTypeStr=single
  Out1 : Outport  OutDataTypeStr=Bus: Obj_Data
  wires:
  Data Type Conversion12/1 -> Bus Creator/13
  Bus Selector/5 -> Data Type Conversion4/1  "<FRS_P1_13_Obj_XAccRel>"
  Bus Selector/8 -> Data Type Conversion7/1  "<FRS_P1_13_Obj_YPos_Stdev>"
  Data Type Conversion15/1 -> Bus Creator/16
  Bus Selector/1 -> Data Type Conversion/1  "<FRS_P1_13_Msg_CheckSum>"
  Bus Selector/15 -> Data Type Conversion14/1  "<FRS_P2_13_Obj_MeasFlag>"
  Bus Selector/3 -> Data Type Conversion2/1  "<FRS_P1_13_Obj_ExstProb>"
  Bus Selector/13 -> Data Type Conversion12/1  "<FRS_P2_13_Msg_CheckSum>"
  Bus Selector/2 -> Data Type Conversion1/1  "<FRS_P1_13_Msg_AliveCounter>"
  Data Type Conversion11/1 -> Bus Creator/12
  Data Type Conversion5/1 -> Bus Creator/6
  Bus Selector/4 -> Data Type Conversion3/1  "<FRS_P1_13_Obj_XVelRel_Stdev>"
  Bus Selector/7 -> Data Type Conversion6/1  "<FRS_P1_13_Obj_MotionPattern>"
  Data Type Conversion9/1 -> Bus Creator/10
  Bus Selector/6 -> Data Type Conversion5/1  "<FRS_P1_13_Obj_ObstacleProb>"
  Data Type Conversion18/1 -> Bus Creator/19
  Bus Selector/11 -> Data Type Conversion10/1  "<FRS_P1_13_Obj_UpdateFlag>"
  Data Type Conversion17/1 -> Bus Creator/18
  Bus Selector/16 -> Data Type Conversion15/1  "<FRS_P2_13_Obj_YVelRel>"
  Data Type Conversion6/1 -> Bus Creator/7
  Bus Selector/12 -> Data Type Conversion11/1  "<FRS_P1_13_Obj_ID>"
  Data Type Conversion16/1 -> Bus Creator/17
  Bus Selector/9 -> Data Type Conversion8/1  "<FRS_P1_13_Obj_ValidFlag>"
  Bus Selector/17 -> Data Type Conversion16/1  "<FRS_P2_13_Obj_Type>"
  Bus Selector/10 -> Data Type Conversion9/1  "<FRS_P1_13_Obj_XPos_Stdev>"
  Data Type Conversion10/1 -> Bus Creator/11
  Bus Selector/14 -> Data Type Conversion13/1  "<FRS_P2_13_Msg_AliveCounter>"
  Bus Selector/19 -> Data Type Conversion18/1  "<FRS_P2_13_Obj_YPos>"
  Bus Selector/18 -> Data Type Conversion17/1  "<FRS_P2_13_Obj_XPos>"
  Bus Selector/20 -> Data Type Conversion19/1  "<FRS_P2_13_Obj_XVelRel>"
  In1/1 -> Bus Selector/1
  Bus Creator/1 -> Out1/1
  Data Type Conversion/1 -> Bus Creator/1
  Data Type Conversion2/1 -> Bus Creator/3
  Data Type Conversion13/1 -> Bus Creator/14
  Data Type Conversion1/1 -> Bus Creator/2
  Data Type Conversion4/1 -> Bus Creator/5
  Data Type Conversion3/1 -> Bus Creator/4
  Data Type Conversion7/1 -> Bus Creator/8
  Data Type Conversion8/1 -> Bus Creator/9
  Data Type Conversion14/1 -> Bus Creator/15
  Data Type Conversion19/1 -> Bus Creator/20

== system Intergration/Radar410_RX/Subsystem41/Subsystem14 ==
  In1 : Inport
  Bus Creator : BusCreator  Inputs=20  OutDataTypeStr=Bus: Obj_Data  NonVirtualBus=on
      settings: InheritFromInputs=off
  Bus Selector : BusSelector  OutputSignals=FRS_P1_22_Msg_CheckSum,FRS_P1_22_Msg_AliveCounter,FRS_P1_22_Obj_ExstProb,FRS_P1_22_Obj_XVelRel_Stdev,FRS_P1_22_Obj_XAccRel,FRS_P1_22_Obj_ObstacleProb,FRS_P1_22_Obj_MotionPattern,FRS_P1_22_Obj_YPos_Stdev,FRS_P1_22_Obj_ValidFlag,FRS_P1_22_Obj_XPos_Stdev,FRS_P1_22_Obj_UpdateFlag,FRS_P1_22_Obj_ID,FRS_P2_22_Msg_CheckSum,FRS_P2_22_Msg_AliveCounter,FRS_P2_22_Obj_MeasFlag,FRS_P2_22_Obj_YVelRel,FRS_P2_22_Obj_Type,FRS_P2_22_Obj_XPos,FRS_P2_22_Obj_YPos,FRS_P2_22_Obj_XVelRel
  Data Type Conversion{,1..19} (20 alike) : DataTypeConversion  OutDataTypeStr=single
  Out1 : Outport  OutDataTypeStr=Bus: Obj_Data
  wires:
  Data Type Conversion12/1 -> Bus Creator/13
  Bus Selector/5 -> Data Type Conversion4/1  "<FRS_P1_22_Obj_XAccRel>"
  Bus Selector/8 -> Data Type Conversion7/1  "<FRS_P1_22_Obj_YPos_Stdev>"
  Data Type Conversion15/1 -> Bus Creator/16
  Bus Selector/1 -> Data Type Conversion/1  "<FRS_P1_22_Msg_CheckSum>"
  Bus Selector/15 -> Data Type Conversion14/1  "<FRS_P2_22_Obj_MeasFlag>"
  Bus Selector/3 -> Data Type Conversion2/1  "<FRS_P1_22_Obj_ExstProb>"
  Bus Selector/13 -> Data Type Conversion12/1  "<FRS_P2_22_Msg_CheckSum>"
  Bus Selector/2 -> Data Type Conversion1/1  "<FRS_P1_22_Msg_AliveCounter>"
  Data Type Conversion11/1 -> Bus Creator/12
  Data Type Conversion5/1 -> Bus Creator/6
  Bus Selector/4 -> Data Type Conversion3/1  "<FRS_P1_22_Obj_XVelRel_Stdev>"
  Bus Selector/7 -> Data Type Conversion6/1  "<FRS_P1_22_Obj_MotionPattern>"
  Data Type Conversion9/1 -> Bus Creator/10
  Bus Selector/6 -> Data Type Conversion5/1  "<FRS_P1_22_Obj_ObstacleProb>"
  Data Type Conversion18/1 -> Bus Creator/19
  Bus Selector/11 -> Data Type Conversion10/1  "<FRS_P1_22_Obj_UpdateFlag>"
  Data Type Conversion17/1 -> Bus Creator/18
  Bus Selector/16 -> Data Type Conversion15/1  "<FRS_P2_22_Obj_YVelRel>"
  Data Type Conversion6/1 -> Bus Creator/7
  Bus Selector/12 -> Data Type Conversion11/1  "<FRS_P1_22_Obj_ID>"
  Data Type Conversion16/1 -> Bus Creator/17
  Bus Selector/9 -> Data Type Conversion8/1  "<FRS_P1_22_Obj_ValidFlag>"
  Bus Selector/17 -> Data Type Conversion16/1  "<FRS_P2_22_Obj_Type>"
  Bus Selector/10 -> Data Type Conversion9/1  "<FRS_P1_22_Obj_XPos_Stdev>"
  Data Type Conversion10/1 -> Bus Creator/11
  Bus Selector/14 -> Data Type Conversion13/1  "<FRS_P2_22_Msg_AliveCounter>"
  Bus Selector/19 -> Data Type Conversion18/1  "<FRS_P2_22_Obj_YPos>"
  Bus Selector/18 -> Data Type Conversion17/1  "<FRS_P2_22_Obj_XPos>"
  Bus Selector/20 -> Data Type Conversion19/1  "<FRS_P2_22_Obj_XVelRel>"
  In1/1 -> Bus Selector/1
  Bus Creator/1 -> Out1/1
  Data Type Conversion/1 -> Bus Creator/1
  Data Type Conversion2/1 -> Bus Creator/3
  Data Type Conversion13/1 -> Bus Creator/14
  Data Type Conversion1/1 -> Bus Creator/2
  Data Type Conversion4/1 -> Bus Creator/5
  Data Type Conversion3/1 -> Bus Creator/4
  Data Type Conversion7/1 -> Bus Creator/8
  Data Type Conversion8/1 -> Bus Creator/9
  Data Type Conversion14/1 -> Bus Creator/15
  Data Type Conversion19/1 -> Bus Creator/20
